simulink model "test2"  (Simulink 9.2)
settings: Solver=VariableStepAuto  StartTime=0.0  StopTime=20  RelTol=1e-3
libraries: Solver_SF x1
settings Model: Creator=KZX  LastModifiedBy=孙重豪
settings DataIOCC: LimitDataPoints=off  SaveFormat=Dataset  SignalLoggingSaveFormat=Dataset
settings OptimizationCC: LifeSpan=auto
settings DebuggingCC: UnderspecifiedInitializationDetection=Simplified  MergeDetectMultiDrivingBlocksExec=error  FcnCallInpInsideContextMsg=error  StateNameClashWarn=none  SFUnexpectedBacktrackingDiag=error  SFNoUnconditionalDefaultTransitionDiag=error  SFExecutionAtInitializationDiag=warning
settings HardwareCC: ProdBitPerPointer=64  ProdBitPerSizeT=64  ProdBitPerPtrDiffT=64  ProdLargestAtomicFloat=Float  ProdIntDivRoundTo=Zero  ProdEndianess=LittleEndian  ProdWordSize=64  ProdHWDeviceType=Intel->x86-64 (Windows64)
settings ModelReferenceCC: PropagateSignalLabelsOutOfModel=on
settings SFSimCC: SimUseLocalCustomCode=on
settings RTWCC: RTWUseLocalCustomCode=on
settings CodeAppCC: StateflowObjectComments=off
settings GRTTargetCC: TargetLangStandard=C99 (ISO)  GeneratePreprocessorConditionals=Use local settings  CombineOutputUpdateFcns=on  GRTInterface=off
settings ConfigComp: CovMetricSettings=dwe  CovHtmlReporting=off  CovSaveCumulativeToWorkspaceVar=off  CovSaveSingleToWorkspaceVar=off  CovExternalEMLEnable=on

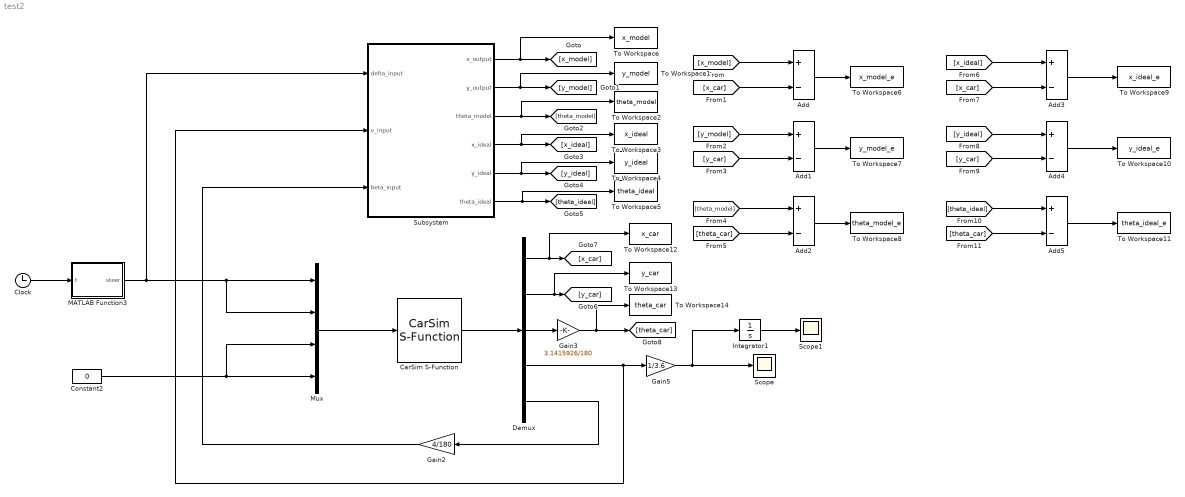
== system test2 ==
  Add{,1..5} (6 alike) : Sum  Inputs=+-
  CarSim S-Function : Solver_SF/CarSim S-Function  Priority=1  SIMFILE=simfile.sim
  Clock : Clock
  Constant2 : Constant  Value=0
  Demux : Demux  Outputs=5
  Gain2 : Gain  Gain=4/180
  Gain3 : Gain  Gain=3.1415926/180
  Gain5 : Gain  Gain=1/3.6
  Integrator1 : Integrator
  MATLAB Function3 : MATLAB Function  TreatAsAtomicUnit=on
  Mux : Mux
  Scope : Scope
  Scope1 : Scope
  Subsystem : Subsystem
  To Workspace : ToWorkspace  VariableName=x_model  SaveFormat=Timeseries  SampleTime=-1
  To Workspace1 : ToWorkspace  VariableName=y_model  SaveFormat=Timeseries  SampleTime=-1
  To Workspace10 : ToWorkspace  VariableName=y_ideal_e  SaveFormat=Timeseries  SampleTime=-1
  To Workspace11 : ToWorkspace  VariableName=theta_ideal_e  SaveFormat=Timeseries  SampleTime=-1
  To Workspace12 : ToWorkspace  VariableName=x_car  SaveFormat=Timeseries  SampleTime=-1
  To Workspace13 : ToWorkspace  VariableName=y_car  SaveFormat=Timeseries  SampleTime=-1
  To Workspace14 : ToWorkspace  VariableName=theta_car  SaveFormat=Timeseries  SampleTime=-1
  To Workspace2 : ToWorkspace  VariableName=theta_model  SaveFormat=Timeseries  SampleTime=-1
  To Workspace3 : ToWorkspace  VariableName=x_ideal  SaveFormat=Timeseries  SampleTime=-1
  To Workspace4 : ToWorkspace  VariableName=y_ideal  SaveFormat=Timeseries  SampleTime=-1
  To Workspace5 : ToWorkspace  VariableName=theta_ideal  SaveFormat=Timeseries  SampleTime=-1
  To Workspace6 : ToWorkspace  VariableName=x_model_e  SaveFormat=Timeseries  SampleTime=-1
  To Workspace7 : ToWorkspace  VariableName=y_model_e  SaveFormat=Timeseries  SampleTime=-1
  To Workspace8 : ToWorkspace  VariableName=theta_model_e  SaveFormat=Timeseries  SampleTime=-1
  To Workspace9 : ToWorkspace  VariableName=x_ideal_e  SaveFormat=Timeseries  SampleTime=-1
  wires:
  [x_car] -> Add3/2
  [x_model] -> Add/1
  Demux/3 -> Gain3/1
  Add2/1 -> To Workspace8/1
  Gain3/1 -> To Workspace14/1, [theta_car]
  Subsystem/5(y_ideal) -> To Workspace4/1, [y_ideal]
  Add/1 -> To Workspace6/1
  [theta_model] -> Add2/1
  Add1/1 -> To Workspace7/1
  Gain5/1 -> Scope/1, Integrator1/1
  Subsystem/4(x_ideal) -> To Workspace3/1, [x_ideal]
  [y_ideal] -> Add4/1
  [x_car] -> Add/2
  Demux/1 -> To Workspace12/1, [x_car]
  Subsystem/6(theta_ideal) -> To Workspace5/1, [theta_ideal]
  Demux/2 -> To Workspace13/1, [y_car]
  [y_car] -> Add4/2
  [theta_ideal] -> Add5/1
  Add4/1 -> To Workspace10/1
  Add3/1 -> To Workspace9/1
  MATLAB Function3/1(steer) -> Mux/1, Mux/2, Subsystem/1(delta_input)
  Subsystem/2(y_output) -> To Workspace1/1, [y_model]
  Subsystem/3(theta_model) -> To Workspace2/1, [theta_model]
  Demux/5 -> Gain2/1
  Constant2/1 -> Mux/3, Mux/4
  Add5/1 -> To Workspace11/1
  Subsystem/1(x_output) -> To Workspace/1, [x_model]
  CarSim S-Function/1 -> Demux/1
  Integrator1/1 -> Scope1/1
  [y_car] -> Add1/2
  [theta_car] -> Add2/2
  [theta_car] -> Add5/2
  [y_model] -> Add1/1
  Demux/4 -> Gain5/1, Subsystem/2(v_input)
  Mux/1 -> CarSim S-Function/1
  Clock/1 -> MATLAB Function3/1(t)
  Gain2/1 -> Subsystem/3(beta_input)
  [x_ideal] -> Add3/1

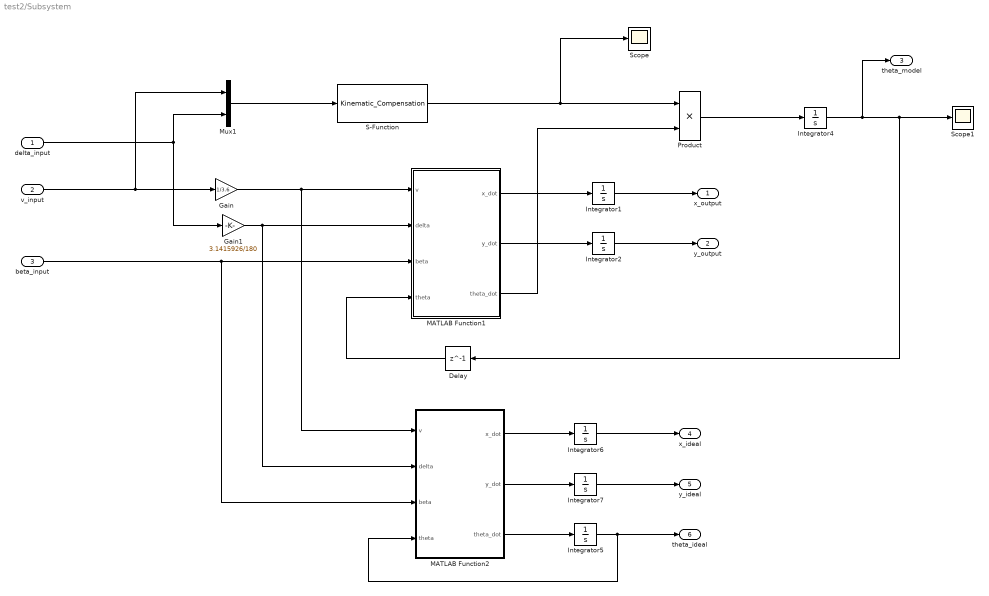
== system test2/Subsystem ==
  delta_input : Inport
  v_input : Inport  Port=2
  beta_input : Inport  Port=3
  Delay : Delay  DelayLength=1
  Gain : Gain  Gain=1/3.6
  Gain1 : Gain  Gain=3.1415926/180
  Integrator{1..2,4..7} (6 alike) : Integrator
  MATLAB Function1 : MATLAB Function  TreatAsAtomicUnit=on
  MATLAB Function2 : MATLAB Function  TreatAsAtomicUnit=on
  Mux1 : Mux  Inputs=2
  Product : Product
  S-Function : S-Function  FunctionName=Kinematic_Compensation  SFunctionModules='1'  SFunctionDeploymentMode=off  EnableBusSupport=off
  Scope : Scope
  Scope1 : Scope
  x_output : Outport
  y_output : Outport  Port=2
  theta_model : Outport  Port=3
  x_ideal : Outport  Port=4
  y_ideal : Outport  Port=5
  theta_ideal : Outport  Port=6
  wires:
  Gain1/1 -> MATLAB Function1/2(delta), MATLAB Function2/2(delta)
  Product/1 -> Integrator4/1
  v_input/1 -> Mux1/1, Gain/1
  delta_input/1 -> Mux1/2, Gain1/1
  Mux1/1 -> S-Function/1
  Integrator4/1 -> theta_model/1, Delay/1, Scope1/1
  MATLAB Function1/2(y_dot) -> Integrator2/1
  Delay/1 -> MATLAB Function1/4(theta)
  MATLAB Function1/3(theta_dot) -> Product/2
  Gain/1 -> MATLAB Function1/1(v), MATLAB Function2/1(v)
  S-Function/1 -> Scope/1, Product/1
  MATLAB Function1/1(x_dot) -> Integrator1/1
  beta_input/1 -> MATLAB Function1/3(beta), MATLAB Function2/3(beta)
  Integrator1/1 -> x_output/1
  Integrator2/1 -> y_output/1
  MATLAB Function2/3(theta_dot) -> Integrator5/1
  Integrator5/1 -> theta_ideal/1, MATLAB Function2/4(theta)
  MATLAB Function2/1(x_dot) -> Integrator6/1
  MATLAB Function2/2(y_dot) -> Integrator7/1
  Integrator7/1 -> y_ideal/1
  Integrator6/1 -> x_ideal/1

== matlab function Subsystem/MATLAB Function1 ==
  data: v input double; x_dot output double; delta input double; beta input double; theta input double; y_dot output double; theta_dot output double
function [x_dot, y_dot, theta_dot]    = fcn(v, delta,beta,theta)
L = 3.1;
x_dot = v * cos(theta + beta);
y_dot = v * sin(theta + beta);
theta_dot =v * cos(beta) * tan(delta) / L;

== matlab function Subsystem/MATLAB Function2 ==
  data: v input double; x_dot output double; delta input double; beta input double; theta input double; y_dot output double; theta_dot output double
function [x_dot, y_dot, theta_dot]    = fcn(v, delta,beta,theta)
L = 3.1;
x_dot = v * cos(theta + beta);
y_dot = v * sin(theta + beta);
theta_dot =v * cos(beta) * tan(delta) / L;

== matlab function MATLAB Function3 ==
  data: steer output double; t input double
function steer = fcn(t)
% steer =20;
   if  t < 10
       steer = 2.5 * t;
   else
       steer = 25 - 2 * (t - 10);
   end
% steer = 0;
end
